simulink model "RefModel_Ecompass_Set"  (R2020b)
settings: Solver=ode1  StartTime=0.0  StopTime=inf  FixedStep=Ts_Navi.Ts_Base  MaxStep=Ts  RelTol=1e-3  EnableMultiTasking=on
values from neighbouring files (symbols this model uses):
  mag1 = double([Sensors.mag1.mag_x, Sensors.mag1.mag_y, Sensors.mag1.mag_z])    [navi_marg22.m]    (also in navi_marg24.m; navi_mvo17.m)
  mag2 = double([Sensors.mag2.mag_x, Sensors.mag2.mag_y, Sensors.mag2.mag_z])    [navi_marg22.m]    (also in navi_marg24.m; navi_mvo17.m)
undefined symbols (not defined in the file or in its folder): accel_x, accel_y, accel_z, IMU1, IMU2, IMU3, mag_x, mag_y, mag_z, SENSOR_ALIGNMENT_PARAM_V10, SENSOR_ALIGNMENT_PARAM_V1000, SENSOR_ALIGNMENT_PARAM_V10_1
libraries: discretizing x3
settings Model: disc_configurable_lib=RefModel_Ecompass_Set_disc_lib  Creator=sl  LastModifiedBy=sl
settings SolverCC: AutoInsertRateTranBlk=on
settings DataIOCC: SaveOutput=off  SaveTime=off
settings OptimizationCC: DefaultParameterBehavior=Inlined  EnhancedBackFolding=on  PassReuseOutputArgsAs=Individual arguments  ZeroExternalMemoryAtStartup=off  ZeroInternalMemoryAtStartup=off  OptimizeBlockOrder=speed  DifferentSizesBufferReuse=on  OptimizationCustomize=off  EfficientTunableParamExpr=on
settings DebuggingCC: InheritedTsInSrcMsg=none  MultiTaskDSMMsg=warning  ParameterPrecisionLossMsg=none  ParameterTunabilityLossMsg=error  UnconnectedInputMsg=none  UnconnectedOutputMsg=none  UnconnectedLineMsg=none
settings HardwareCC: ProdBitPerPointer=32  ProdBitPerSizeT=32  ProdBitPerPtrDiffT=32  ProdLargestAtomicInteger=Long  ProdLargestAtomicFloat=Double  ProdWordSize=32  ProdHWDeviceType=ARM Compatible->ARM Cortex
settings ModelReferenceCC: ParallelModelReferenceMATLABWorkerInit=Copy Base Workspace  ModelReferenceNumInstancesAllowed=Single
settings SFSimCC: MATLABDynamicMemAlloc=off
settings RTWCC: Description=Embedded Coder  SystemTargetFile=ert.tlc  GenCodeOnly=on  PackageGeneratedCodeAndArtifacts=on  TemplateMakefile=ert_default_tmf  GenerateReport=on  IncludeHyperlinkInReport=on  LaunchReport=on  GenerateTraceInfo=on  GenerateTraceReport=on  GenerateTraceReportSl=on  GenerateTraceReportSf=on  GenerateTraceReportEml=on
settings CodeAppCC: ForceParamTrailComments=on  IgnoreCustomStorageClasses=off  MaxIdLength=64  OperatorAnnotations=on  SimulinkDataObjDesc=on  SFDataObjDesc=on  MATLABFcnDesc=on  InsertBlockDesc=on  MATLABSourceComments=on
settings ERTTargetCC: TargetLangStandard=C99 (ISO)  GenerateSampleERTMain=on  LogVarNameModifier=none  SupportVariableSizeSignals=on  InlinedParameterPlacement=NonHierarchical  ERTCustomFileTemplate=example_file_process.tlc  ERTFilePackagingFormat=Compact

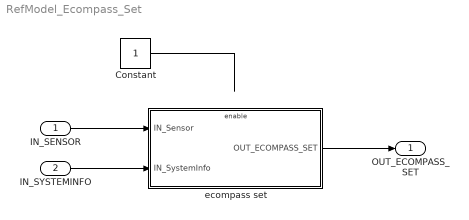
== system RefModel_Ecompass_Set ==
  IN_SENSOR : Inport  OutDataTypeStr=Bus: BUS_SENSOR
  IN_SYSTEMINFO : Inport  Port=2  OutDataTypeStr=Bus: BUS_SYSTEMINFO_INPUT  BusOutputAsStruct=on
  Constant : Constant
  ecompass set : Subsystem
  OUT_ECOMPASS_SET : Outport  OutDataTypeStr=Bus: BUS_NAVI_ECOMPASS_SET
  wires:
  IN_SYSTEMINFO/1 -> ecompass set/2(IN_SystemInfo)
  ecompass set/1(OUT_ECOMPASS_SET) -> OUT_ECOMPASS_SET/1
  Constant/1 -> ?
  IN_SENSOR/1 -> ecompass set/1(IN_Sensor)

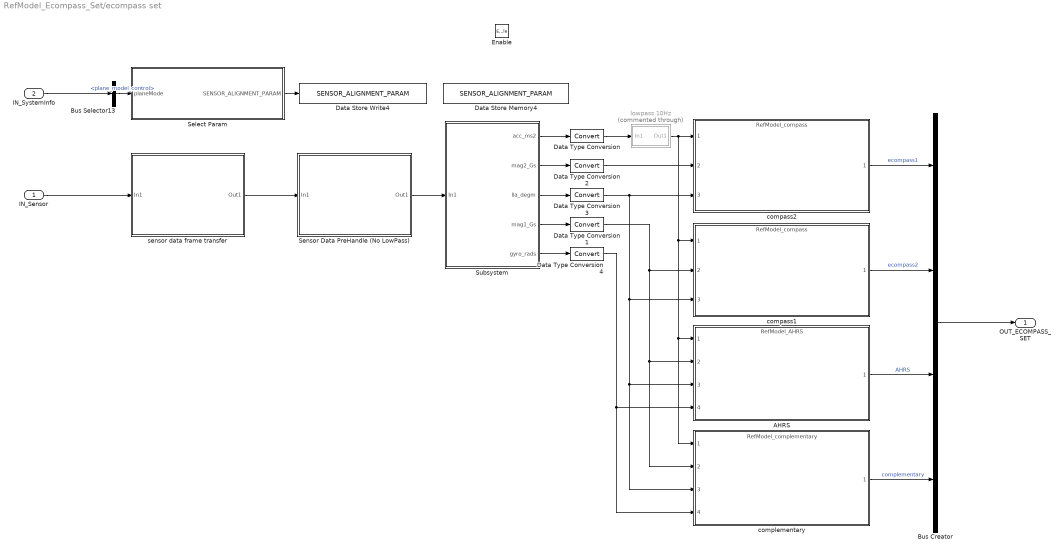
== system RefModel_Ecompass_Set/ecompass set ==
  IN_Sensor : Inport
  IN_SystemInfo : Inport  Port=2  BusOutputAsStruct=on
  Enable : EnablePort
  AHRS : ModelReference  ModelNameDialog=RefModel_AHRS.slx  SimulationMode=Normal  ModelReferenceVersion=2.6
  Bus Creator : BusCreator  Inputs=4
  Bus Selector13 : BusSelector  OutputSignals=plane_model_control
  Data Store Memory4 : DataStoreMemory  DataStoreName=SENSOR_ALIGNMENT_PARAM  ReadBeforeWriteMsg=warning  WriteAfterWriteMsg=warning  WriteAfterReadMsg=warning  ShowAdditionalParam=off  OutDataTypeStr=Bus: BUS_SENSOR_ALIGNMENT_PARAM  Dimensions=1
  Data Store Write4 : DataStoreWrite  DataStoreName=SENSOR_ALIGNMENT_PARAM
  Data Type Conversion{,1..4} (5 alike) : DataTypeConversion
  Select Param : Subsystem
  Sensor Data PreHandle (No LowPass) : Subsystem
  Subsystem : Subsystem
  compass1 : ModelReference  ModelNameDialog=RefModel_compass.slx  SimulationMode=Normal  ModelReferenceVersion=2.3
  compass2 : ModelReference  ModelNameDialog=RefModel_compass.slx  SimulationMode=Normal  ModelReferenceVersion=2.3
  complementary : ModelReference  ModelNameDialog=RefModel_complementary.slx  SimulationMode=Normal  ModelReferenceVersion=2.2
  lowpass 10Hz : Subsystem  Commented=through
  sensor data frame transfer : Subsystem
  OUT_ECOMPASS_SET : Outport
  wires:
  Sensor Data PreHandle (No LowPass)/1(Out1) -> Subsystem/1(In1)
  sensor data frame transfer/1(Out1) -> Sensor Data PreHandle (No LowPass)/1(In1)
  Data Type Conversion/1 -> lowpass 10Hz/1(In1)
  Subsystem/1(acc_ms2) -> Data Type Conversion/1
  Subsystem/2(mag2_Gs) -> Data Type Conversion2/1
  Data Type Conversion2/1 -> compass2/2
  lowpass 10Hz/1(Out1) -> complementary/1, AHRS/1, compass1/1, compass2/1
  Subsystem/4(mag1_Gs) -> Data Type Conversion1/1
  Data Type Conversion4/1 -> complementary/4, AHRS/4
  Data Type Conversion3/1 -> complementary/3, AHRS/3, compass1/3, compass2/3
  Data Type Conversion1/1 -> complementary/2, AHRS/2, compass1/2
  Subsystem/3(lla_degm) -> Data Type Conversion3/1
  Subsystem/5(gyro_rads) -> Data Type Conversion4/1
  AHRS/1 -> Bus Creator/3  "AHRS"
  complementary/1 -> Bus Creator/4  "complementary"
  Bus Creator/1 -> OUT_ECOMPASS_SET/1
  compass2/1 -> Bus Creator/1  "ecompass1"
  compass1/1 -> Bus Creator/2  "ecompass2"
  IN_Sensor/1 -> sensor data frame transfer/1(In1)
  Select Param/1(SENSOR_ALIGNMENT_PARAM) -> Data Store Write4/1
  IN_SystemInfo/1 -> Bus Selector13/1
  Bus Selector13/1 -> Select Param/1(planeMode)  "<plane_model_control>"

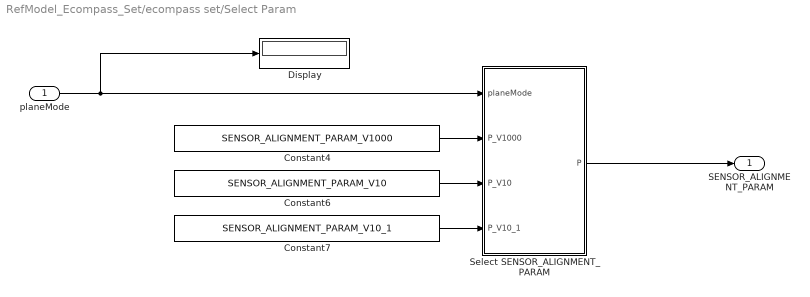
== system RefModel_Ecompass_Set/ecompass set/Select Param ==
  planeMode : Inport
  Constant4 : Constant  Value=SENSOR_ALIGNMENT_PARAM_V1000  OutDataTypeStr=Bus: BUS_SENSOR_ALIGNMENT_PARAM
  Constant6 : Constant  Value=SENSOR_ALIGNMENT_PARAM_V10  OutDataTypeStr=Bus: BUS_SENSOR_ALIGNMENT_PARAM
  Constant7 : Constant  Value=SENSOR_ALIGNMENT_PARAM_V10_1  OutDataTypeStr=Bus: BUS_SENSOR_ALIGNMENT_PARAM
  Display : Display
  Select SENSOR_ALIGNMENT_PARAM : MATLAB Function  TreatAsAtomicUnit=on
  SENSOR_ALIGNMENT_PARAM : Outport
  wires:
  planeMode/1 -> Display/1, Select SENSOR_ALIGNMENT_PARAM/1(planeMode)
  Constant4/1 -> Select SENSOR_ALIGNMENT_PARAM/2(P_V1000)
  Constant6/1 -> Select SENSOR_ALIGNMENT_PARAM/3(P_V10)
  Select SENSOR_ALIGNMENT_PARAM/1(P) -> SENSOR_ALIGNMENT_PARAM/1
  Constant7/1 -> Select SENSOR_ALIGNMENT_PARAM/4(P_V10_1)

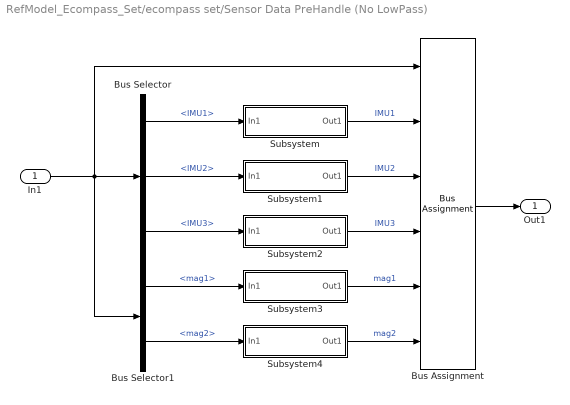
== system RefModel_Ecompass_Set/ecompass set/Sensor Data PreHandle (No LowPass) ==
  In1 : Inport
  Bus Assignment : BusAssignment  AssignedSignals=IMU1,IMU2,IMU3,mag1,mag2
  Bus Selector : BusSelector  OutputSignals=IMU1,IMU2,IMU3
  Bus Selector1 : BusSelector  OutputSignals=mag1,mag2
  Subsystem : Subsystem
  Subsystem1 : Subsystem
  Subsystem2 : Subsystem
  Subsystem3 : Subsystem
  Subsystem4 : Subsystem
  Out1 : Outport
  wires:
  Bus Selector1/2 -> Subsystem4/1(In1)  "<mag2>"
  Bus Selector1/1 -> Subsystem3/1(In1)  "<mag1>"
  Bus Selector/3 -> Subsystem2/1(In1)  "<IMU3>"
  Bus Selector/2 -> Subsystem1/1(In1)  "<IMU2>"
  Bus Selector/1 -> Subsystem/1(In1)  "<IMU1>"
  Subsystem4/1(Out1) -> Bus Assignment/6  "mag2"
  Subsystem3/1(Out1) -> Bus Assignment/5  "mag1"
  In1/1 -> Bus Selector/1, Bus Assignment/1, Bus Selector1/1
  Bus Assignment/1 -> Out1/1
  Subsystem2/1(Out1) -> Bus Assignment/4  "IMU3"
  Subsystem1/1(Out1) -> Bus Assignment/3  "IMU2"
  Subsystem/1(Out1) -> Bus Assignment/2  "IMU1"

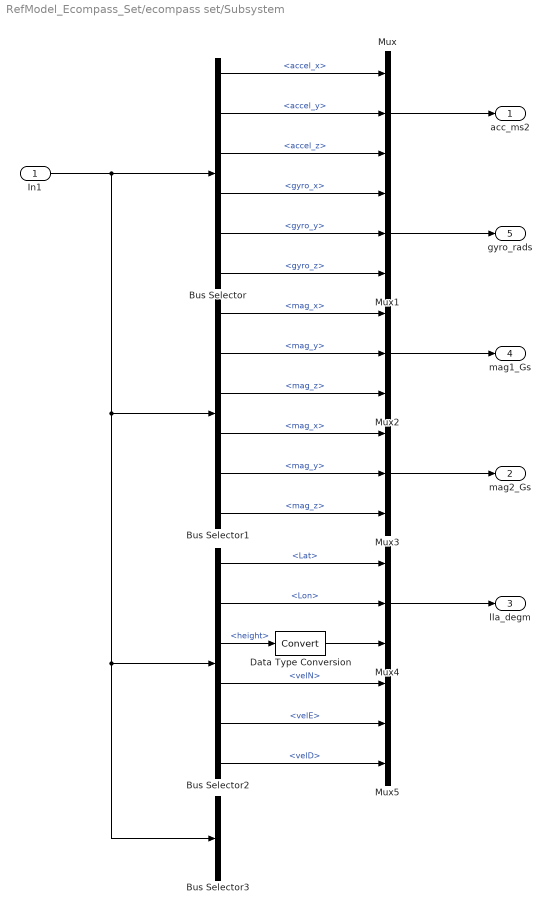
== system RefModel_Ecompass_Set/ecompass set/Subsystem ==
  In1 : Inport
  Bus Selector : BusSelector  OutputSignals=IMU1.accel_x,IMU1.accel_y,IMU1.accel_z,IMU1.gyro_x,IMU1.gyro_y,IMU1.gyro_z
  Bus Selector1 : BusSelector  OutputSignals=mag1.mag_x,mag1.mag_y,mag1.mag_z,mag2.mag_x,mag2.mag_y,mag2.mag_z
  Bus Selector2 : BusSelector  OutputSignals=ublox1.Lat,ublox1.Lon,ublox1.height,ublox1.velN,ublox1.velE,ublox1.velD
  Bus Selector3 : BusSelector  OutputSignals=baro1.alt_baro,radar1.Range
  Data Type Conversion : DataTypeConversion
  Mux{,1..5} (6 alike) : Mux  Inputs=3
  acc_ms2 : Outport
  mag2_Gs : Outport  Port=2
  lla_degm : Outport  Port=3
  mag1_Gs : Outport  Port=4
  gyro_rads : Outport  Port=5
  wires:
  In1/1 -> Bus Selector3/1, Bus Selector2/1, Bus Selector1/1, Bus Selector/1
  Bus Selector/1 -> Mux/1  "<accel_x>"
  Bus Selector/2 -> Mux/2  "<accel_y>"
  Bus Selector/3 -> Mux/3  "<accel_z>"
  Bus Selector/4 -> Mux1/1  "<gyro_x>"
  Bus Selector/5 -> Mux1/2  "<gyro_y>"
  Bus Selector/6 -> Mux1/3  "<gyro_z>"
  Mux/1 -> acc_ms2/1
  Bus Selector1/1 -> Mux2/1  "<mag_x>"
  Bus Selector1/2 -> Mux2/2  "<mag_y>"
  Bus Selector1/3 -> Mux2/3  "<mag_z>"
  Bus Selector1/4 -> Mux3/1  "<mag_x>"
  Bus Selector1/5 -> Mux3/2  "<mag_y>"
  Bus Selector1/6 -> Mux3/3  "<mag_z>"
  Bus Selector2/6 -> Mux5/3  "<velD>"
  Bus Selector2/5 -> Mux5/2  "<velE>"
  Bus Selector2/4 -> Mux5/1  "<velN>"
  Bus Selector2/3 -> Data Type Conversion/1  "<height>"
  Bus Selector2/2 -> Mux4/2  "<Lon>"
  Bus Selector2/1 -> Mux4/1  "<Lat>"
  Mux4/1 -> lla_degm/1
  Data Type Conversion/1 -> Mux4/3
  Mux3/1 -> mag2_Gs/1
  Mux2/1 -> mag1_Gs/1
  Mux1/1 -> gyro_rads/1

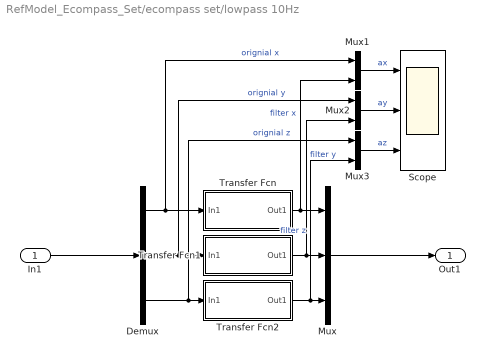
== system RefModel_Ecompass_Set/ecompass set/lowpass 10Hz ==
  In1 : Inport
  Demux : Demux  Outputs=3
  Mux : Mux  Inputs=3
  Mux1 : Mux  Inputs=2
  Mux2 : Mux  Inputs=2
  Mux3 : Mux  Inputs=2
  Scope : Scope  NumInputPorts=3
  Transfer Fcn : Subsystem  BlockChoice=Transfer Fcn discrete version 1
      settings: MemberBlocks=Transfer Fcn,Transfer Fcn discrete version 1
      settings: TemplateBlock=|
      | RefModel_Ecompass_Set_disc_lib/Transfer Fcn
      | (Configurable Subsystem)
  Transfer Fcn1 : Subsystem  BlockChoice=Transfer Fcn1 discrete version 1
      settings: MemberBlocks=Transfer Fcn1,Transfer Fcn1 discrete version 1
      settings: TemplateBlock=|
      | RefModel_Ecompass_Set_disc_lib/Transfer Fcn1
      | (Configurable Subsystem)
  Transfer Fcn2 : Subsystem  BlockChoice=Transfer Fcn2 discrete version 1
      settings: MemberBlocks=Transfer Fcn2,Transfer Fcn2 discrete version 1
      settings: TemplateBlock=|
      | RefModel_Ecompass_Set_disc_lib/Transfer Fcn2
      | (Configurable Subsystem)
  Out1 : Outport
  wires:
  In1/1 -> Demux/1
  Demux/1 -> Mux1/1, Transfer Fcn/1(In1)  "orignial x"
  Demux/2 -> Mux2/1, Transfer Fcn1/1(In1)  "orignial y"
  Mux/1 -> Out1/1
  Transfer Fcn1/1(Out1) -> Mux2/2, Mux/2  "filter y"
  Transfer Fcn2/1(Out1) -> Mux3/2, Mux/3  "filter z"
  Transfer Fcn/1(Out1) -> Mux1/2, Mux/1  "filter x"
  Demux/3 -> Mux3/1, Transfer Fcn2/1(In1)  "orignial z"
  Mux1/1 -> Scope/1  "ax"
  Mux2/1 -> Scope/2  "ay"
  Mux3/1 -> Scope/3  "az"

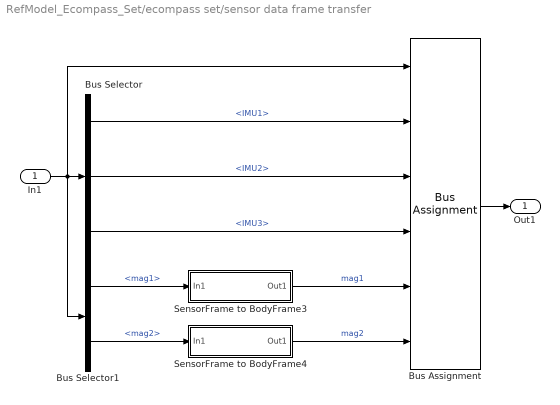
== system RefModel_Ecompass_Set/ecompass set/sensor data frame transfer ==
  In1 : Inport
  Bus Assignment : BusAssignment  AssignedSignals=IMU1,IMU2,IMU3,mag1,mag2
  Bus Selector : BusSelector  OutputSignals=IMU1,IMU2,IMU3
  Bus Selector1 : BusSelector  OutputSignals=mag1,mag2
  SensorFrame to BodyFrame3 : Subsystem
  SensorFrame to BodyFrame4 : Subsystem
  Out1 : Outport
  wires:
  Bus Selector/1 -> Bus Assignment/2  "<IMU1>"
  Bus Selector/2 -> Bus Assignment/3  "<IMU2>"
  Bus Selector/3 -> Bus Assignment/4  "<IMU3>"
  Bus Assignment/1 -> Out1/1
  In1/1 -> Bus Selector1/1, Bus Assignment/1, Bus Selector/1
  Bus Selector1/1 -> SensorFrame to BodyFrame3/1(In1)  "<mag1>"
  Bus Selector1/2 -> SensorFrame to BodyFrame4/1(In1)  "<mag2>"
  SensorFrame to BodyFrame3/1(Out1) -> Bus Assignment/5  "mag1"
  SensorFrame to BodyFrame4/1(Out1) -> Bus Assignment/6  "mag2"

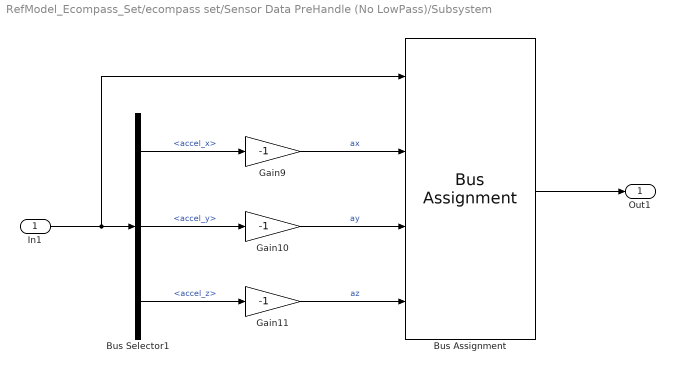
== system RefModel_Ecompass_Set/ecompass set/Sensor Data PreHandle (No LowPass)/Subsystem ==
  In1 : Inport
  Bus Assignment : BusAssignment  AssignedSignals=accel_x,accel_y,accel_z
  Bus Selector1 : BusSelector  OutputSignals=accel_x,accel_y,accel_z
  Gain10 : Gain  Gain=-1
  Gain11 : Gain  Gain=-1
  Gain9 : Gain  Gain=-1
  Out1 : Outport
  wires:
  Bus Selector1/3 -> Gain11/1  "<accel_z>"
  In1/1 -> Bus Assignment/1, Bus Selector1/1
  Bus Selector1/2 -> Gain10/1  "<accel_y>"
  Bus Selector1/1 -> Gain9/1  "<accel_x>"
  Gain9/1 -> Bus Assignment/2  "ax"
  Gain10/1 -> Bus Assignment/3  "ay"
  Gain11/1 -> Bus Assignment/4  "az"
  Bus Assignment/1 -> Out1/1

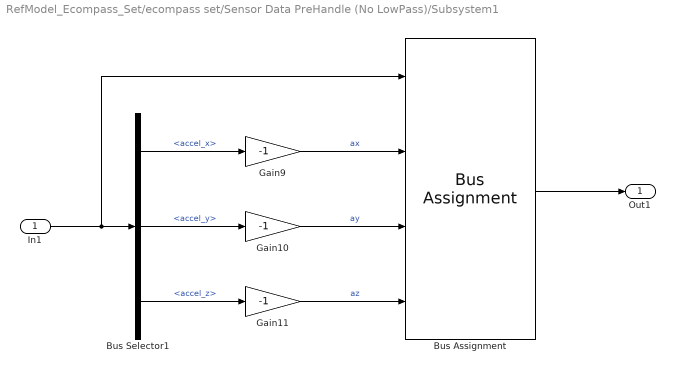
== system RefModel_Ecompass_Set/ecompass set/Sensor Data PreHandle (No LowPass)/Subsystem1 ==
  In1 : Inport
  Bus Assignment : BusAssignment  AssignedSignals=accel_x,accel_y,accel_z
  Bus Selector1 : BusSelector  OutputSignals=accel_x,accel_y,accel_z
  Gain10 : Gain  Gain=-1
  Gain11 : Gain  Gain=-1
  Gain9 : Gain  Gain=-1
  Out1 : Outport
  wires:
  Bus Assignment/1 -> Out1/1
  Gain11/1 -> Bus Assignment/4  "az"
  Gain10/1 -> Bus Assignment/3  "ay"
  Gain9/1 -> Bus Assignment/2  "ax"
  Bus Selector1/1 -> Gain9/1  "<accel_x>"
  Bus Selector1/2 -> Gain10/1  "<accel_y>"
  In1/1 -> Bus Selector1/1, Bus Assignment/1
  Bus Selector1/3 -> Gain11/1  "<accel_z>"

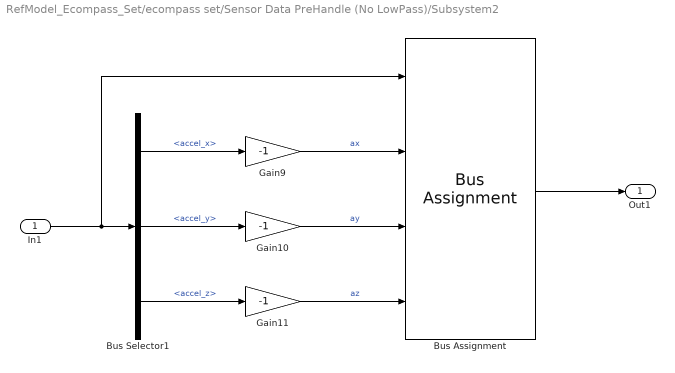
== system RefModel_Ecompass_Set/ecompass set/Sensor Data PreHandle (No LowPass)/Subsystem2 ==
  In1 : Inport
  Bus Assignment : BusAssignment  AssignedSignals=accel_x,accel_y,accel_z
  Bus Selector1 : BusSelector  OutputSignals=accel_x,accel_y,accel_z
  Gain10 : Gain  Gain=-1
  Gain11 : Gain  Gain=-1
  Gain9 : Gain  Gain=-1
  Out1 : Outport
  wires:
  Bus Selector1/3 -> Gain11/1  "<accel_z>"
  In1/1 -> Bus Assignment/1, Bus Selector1/1
  Bus Selector1/2 -> Gain10/1  "<accel_y>"
  Bus Selector1/1 -> Gain9/1  "<accel_x>"
  Gain9/1 -> Bus Assignment/2  "ax"
  Gain10/1 -> Bus Assignment/3  "ay"
  Gain11/1 -> Bus Assignment/4  "az"
  Bus Assignment/1 -> Out1/1

== system RefModel_Ecompass_Set/ecompass set/Sensor Data PreHandle (No LowPass)/Subsystem3 ==
  In1 : Inport
  Bus Assignment : BusAssignment  AssignedSignals=mag_x,mag_y,mag_z
  Bus Selector : BusSelector  OutputSignals=mag_x,mag_y,mag_z
  Gs to uT1 : Gain  Gain=100
  Gs to uT2 : Gain  Gain=100
  Gs to uT3 : Gain  Gain=100
  Out1 : Outport
  wires:
  Bus Selector/3 -> Gs to uT3/1  "<mag_z>"
  Bus Selector/2 -> Gs to uT2/1  "<mag_y>"
  Bus Selector/1 -> Gs to uT1/1  "<mag_x>"
  In1/1 -> Bus Assignment/1, Bus Selector/1
  Gs to uT1/1 -> Bus Assignment/2  "mag_x"
  Gs to uT2/1 -> Bus Assignment/3  "mag_y"
  Gs to uT3/1 -> Bus Assignment/4  "mag_z"
  Bus Assignment/1 -> Out1/1

== system RefModel_Ecompass_Set/ecompass set/Sensor Data PreHandle (No LowPass)/Subsystem4 ==
  In1 : Inport
  Bus Assignment : BusAssignment  AssignedSignals=mag_x,mag_y,mag_z
  Bus Selector : BusSelector  OutputSignals=mag_x,mag_y,mag_z
  Gs to uT1 : Gain  Gain=100
  Gs to uT2 : Gain  Gain=100
  Gs to uT3 : Gain  Gain=100
  Out1 : Outport
  wires:
  Bus Assignment/1 -> Out1/1
  Gs to uT3/1 -> Bus Assignment/4  "mag_z"
  Gs to uT2/1 -> Bus Assignment/3  "mag_y"
  Gs to uT1/1 -> Bus Assignment/2  "mag_x"
  In1/1 -> Bus Selector/1, Bus Assignment/1
  Bus Selector/1 -> Gs to uT1/1  "<mag_x>"
  Bus Selector/2 -> Gs to uT2/1  "<mag_y>"
  Bus Selector/3 -> Gs to uT3/1  "<mag_z>"

== system RefModel_Ecompass_Set/ecompass set/lowpass 10Hz/Transfer Fcn ==
  In1 : Inport
  Transfer Fcn discrete version 1 : discretizing/Discretized Transfer Fcn  Numerator=[1]  Denominator=[.1 1]  AbsTol=auto  SampleTime=0.012  method=zoh  Wc=1
      settings: SourceProductBaseCode=SL
  Out1 : Outport
  wires:
  In1/1 -> Transfer Fcn discrete version 1/1
  Transfer Fcn discrete version 1/1 -> Out1/1

== system RefModel_Ecompass_Set/ecompass set/lowpass 10Hz/Transfer Fcn1 ==
  In1 : Inport
  Transfer Fcn1 discrete version 1 : discretizing/Discretized Transfer Fcn  Numerator=[1]  Denominator=[.1 1]  AbsTol=auto  SampleTime=0.012  method=zoh  Wc=1
      settings: SourceProductBaseCode=SL
  Out1 : Outport
  wires:
  In1/1 -> Transfer Fcn1 discrete version 1/1
  Transfer Fcn1 discrete version 1/1 -> Out1/1

== system RefModel_Ecompass_Set/ecompass set/lowpass 10Hz/Transfer Fcn2 ==
  In1 : Inport
  Transfer Fcn2 discrete version 1 : discretizing/Discretized Transfer Fcn  Numerator=[1]  Denominator=[.1 1]  AbsTol=auto  SampleTime=0.012  method=zoh  Wc=1
      settings: SourceProductBaseCode=SL
  Out1 : Outport
  wires:
  In1/1 -> Transfer Fcn2 discrete version 1/1
  Transfer Fcn2 discrete version 1/1 -> Out1/1

== system RefModel_Ecompass_Set/ecompass set/sensor data frame transfer/SensorFrame to BodyFrame3 ==
  In1 : Inport
  Bus Creator : BusCreator  Inputs=5
  Bus Selector : BusSelector  OutputSignals=time,mag_x,mag_y,mag_z,nChange
  Frame Transfer : Subsystem
  Out1 : Outport
  wires:
  Frame Transfer/3(Out3) -> Bus Creator/4  "mag_z"
  Frame Transfer/2(Out2) -> Bus Creator/3  "mag_y"
  Frame Transfer/1(Out1) -> Bus Creator/2  "mag_x"
  Bus Selector/4 -> Frame Transfer/3(In3)  "<mag_z>"
  Bus Selector/3 -> Frame Transfer/2(In2)  "<mag_y>"
  Bus Selector/2 -> Frame Transfer/1(In1)  "<mag_x>"
  In1/1 -> Bus Selector/1
  Bus Creator/1 -> Out1/1
  Bus Selector/1 -> Bus Creator/1  "<time>"
  Bus Selector/5 -> Bus Creator/5  "<nChange>"

== system RefModel_Ecompass_Set/ecompass set/sensor data frame transfer/SensorFrame to BodyFrame4 ==
  In1 : Inport
  Bus Creator : BusCreator  Inputs=5
  Bus Selector : BusSelector  OutputSignals=time,mag_x,mag_y,mag_z,nChange
  Frame Transfer : Subsystem
  Out1 : Outport
  wires:
  Bus Selector/1 -> Bus Creator/1  "<time>"
  Bus Creator/1 -> Out1/1
  In1/1 -> Bus Selector/1
  Bus Selector/2 -> Frame Transfer/1(In1)  "<mag_x>"
  Bus Selector/3 -> Frame Transfer/2(In2)  "<mag_y>"
  Bus Selector/4 -> Frame Transfer/3(In3)  "<mag_z>"
  Frame Transfer/1(Out1) -> Bus Creator/2  "mag_x"
  Frame Transfer/2(Out2) -> Bus Creator/3  "mag_y"
  Frame Transfer/3(Out3) -> Bus Creator/4  "mag_z"
  Bus Selector/5 -> Bus Creator/5  "<nChange>"

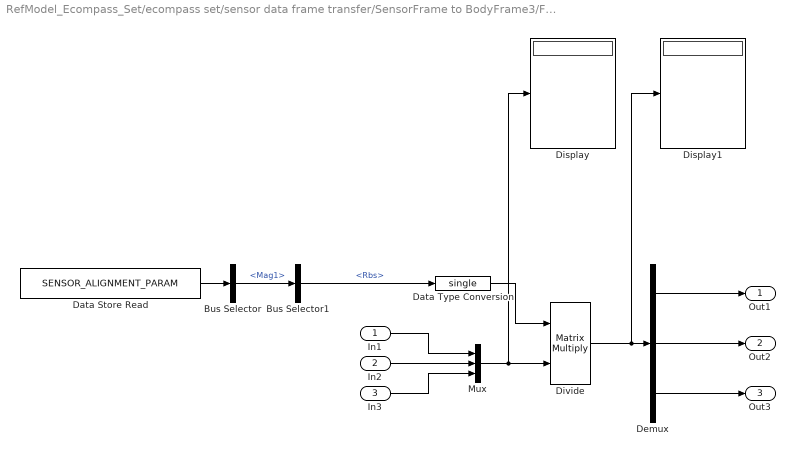
== system RefModel_Ecompass_Set/ecompass set/sensor data frame transfer/SensorFrame to BodyFrame3/Frame Transfer ==
  In1 : Inport
  In2 : Inport  Port=2
  In3 : Inport  Port=3
  Bus Selector : BusSelector  OutputSignals=Mag1
  Bus Selector1 : BusSelector  OutputSignals=Rbs
  Data Store Read : DataStoreRead  DataStoreName=SENSOR_ALIGNMENT_PARAM
  Data Type Conversion : DataTypeConversion  OutDataTypeStr=single
  Demux : Demux  Outputs=3
  Display : Display
  Display1 : Display
  Divide : Product  Inputs=**  Multiplication=Matrix(*)
  Mux : Mux  Inputs=3
  Out1 : Outport
  Out2 : Outport  Port=2
  Out3 : Outport  Port=3
  wires:
  Data Type Conversion/1 -> Divide/1
  Demux/3 -> Out3/1
  Demux/2 -> Out2/1
  Demux/1 -> Out1/1
  Divide/1 -> Demux/1, Display1/1
  Mux/1 -> Divide/2, Display/1
  In3/1 -> Mux/3
  In1/1 -> Mux/1
  In2/1 -> Mux/2
  Bus Selector/1 -> Bus Selector1/1  "<Mag1>"
  Bus Selector1/1 -> Data Type Conversion/1  "<Rbs>"
  Data Store Read/1 -> Bus Selector/1

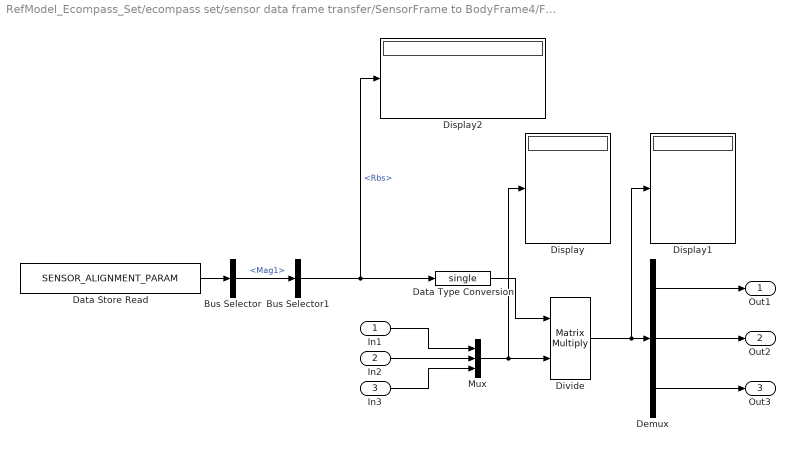
== system RefModel_Ecompass_Set/ecompass set/sensor data frame transfer/SensorFrame to BodyFrame4/Frame Transfer ==
  In1 : Inport
  In2 : Inport  Port=2
  In3 : Inport  Port=3
  Bus Selector : BusSelector  OutputSignals=Mag1
  Bus Selector1 : BusSelector  OutputSignals=Rbs
  Data Store Read : DataStoreRead  DataStoreName=SENSOR_ALIGNMENT_PARAM
  Data Type Conversion : DataTypeConversion  OutDataTypeStr=single
  Demux : Demux  Outputs=3
  Display : Display
  Display1 : Display
  Display2 : Display
  Divide : Product  Inputs=**  Multiplication=Matrix(*)
  Mux : Mux  Inputs=3
  Out1 : Outport
  Out2 : Outport  Port=2
  Out3 : Outport  Port=3
  wires:
  In2/1 -> Mux/2
  In1/1 -> Mux/1
  In3/1 -> Mux/3
  Mux/1 -> Display/1, Divide/2
  Divide/1 -> Display1/1, Demux/1
  Demux/1 -> Out1/1
  Demux/2 -> Out2/1
  Demux/3 -> Out3/1
  Data Type Conversion/1 -> Divide/1
  Bus Selector/1 -> Bus Selector1/1  "<Mag1>"
  Bus Selector1/1 -> Display2/1, Data Type Conversion/1  "<Rbs>"
  Data Store Read/1 -> Bus Selector/1

== matlab function RefModel_Ecompass_Set/ecompass set/Select Param/Select SENSOR_ALIGNMENT_PARAM ==
  data: planeMode input Enum: ENUM_plane_mode; P output Bus: BUS_SENSOR_ALIGNMENT_PARAM; P_V1000 input Bus: BUS_SENSOR_ALIGNMENT_PARAM; P_V10 input Bus: BUS_SENSOR_ALIGNMENT_PARAM; P_V10_1 input Bus: BUS_SENSOR_ALIGNMENT_PARAM
function P = fcn(planeMode,P_V1000,P_V10, P_V10_1)
switch planeMode
    case ENUM_plane_mode.V10
        P = P_V10;
    case {ENUM_plane_mode.V1000,ENUM_plane_mode.V10s}
        P = P_V1000;
    case ENUM_plane_mode.V10_1
        P = P_V10_1;
    otherwise
        P = P_V1000;
end
